simulink model "Copy_of_mcb_bldc_sixstep_f28069mLaunchPad_closeLoop"  (R2023b)
settings: Solver=FixedStepDiscrete  StartTime=0.0  StopTime=2  RelTol=1e-3  EnableMultiTasking=on
InitFcn:
  | mcb_bldc_sixstep_f28069mLaunchPad_data;
values from neighbouring files (symbols this model uses):
  bldc = mcb_SetPMSMMotorParameters('D60MR6430')    [mcb_bldc_sixstep_f28069mLaunchPad_data.m]
  inverter = mcb_SetInverterParameters('SBLMB500')    [mcb_bldc_sixstep_f28069mLaunchPad_data.m]
  PI_params = mcb_SetControllerParameters(bldc,inverter,PU_System,T_pwm,2*Ts,Ts_speed)    [mcb_bldc_sixstep_f28069mLaunchPad_data.m]
  speedRefADCOffset = 44    [mcb_bldc_sixstep_f28069mLaunchPad_data.m]
  target = mcb_SetProcessorDetails('F28069M',PWM_frequency)    [mcb_bldc_sixstep_f28069mLaunchPad_data.m]
  Ts = 0.03    [dataMonitoringArr.m]    (also in mcb_bldc_sixstep_f28069mLaunchPad_data.m = 5e-05)
  Ts_speed = 10*Ts    (= 0.0005)    [mcb_bldc_sixstep_f28069mLaunchPad_data.m]
undefined symbols (not defined in the file or in its folder): Down, GPTRIP1SEL, GPTRIP2SEL, TZ1, TZ2, Up
libraries: c2802xlib x8, c2806xlib x6, c280xlib x5, mcbcontrolslib x3, mcbpositiondecoderlib x3, slpidlib x2, simulink x2, svdschedulerlib x1
(part 2 of 2)

== system Copy_of_mcb_bldc_sixstep_f28069mLaunchPad_closeLoop/Current Control/Data_Logging/Data_Conditioning ==
  In1 : Inport
  Data Type Conversion : DataTypeConversion  OutDataTypeStr=fixdt(1,16,12)  RndMeth=Simplest  SaturateOnIntegerOverflow=off
  Data Type Conversion3 : DataTypeConversion  OutDataTypeStr=uint16  ConvertRealWorld=Stored Integer (SI)  SaturateOnIntegerOverflow=off  RndMeth=Floor
  Out1 : Outport  VectorParamsAs1DForOutWhenUnconnected=off
  wires:
  In1/1 -> Data Type Conversion/1
  Data Type Conversion3/1 -> Out1/1
  Data Type Conversion/1 -> Data Type Conversion3/1

== system Copy_of_mcb_bldc_sixstep_f28069mLaunchPad_closeLoop/Current Control/Data_Logging/End ==
  Data : Inport
  Data_width : Inport  Port=2
  Action Port : ActionPort  ActionPortLabel=elseif(u1 == 599)
  Bias : Bias  Bias=1  SaturateOnIntegerOverflow=off
  Mux : Mux  Inputs=2
  Start : Constant  Value=hex2dec('4545')  OutDataTypeStr=uint16
  Data_out : Outport  VectorParamsAs1DForOutWhenUnconnected=off
  Iteration : Outport  Port=2  VectorParamsAs1DForOutWhenUnconnected=off
  wires:
  Mux/1 -> Data_out/1
  Data_width/1 -> Bias/1
  Start/1 -> Mux/2
  Bias/1 -> Iteration/1
  Data/1 -> Mux/1

== system Copy_of_mcb_bldc_sixstep_f28069mLaunchPad_closeLoop/Current Control/Data_Logging/Start ==
  Data : Inport
  Data_width : Inport  Port=2
  Action Port : ActionPort  ActionPortLabel=if(u1 == 0)
  Bias : Bias  Bias=1  SaturateOnIntegerOverflow=off
  End : Constant  Value=hex2dec('5353')  OutDataTypeStr=uint16
  Mux : Mux  Inputs=2
  Data_out : Outport  VectorParamsAs1DForOutWhenUnconnected=off
  Iteration : Outport  Port=2  VectorParamsAs1DForOutWhenUnconnected=off
  wires:
  End/1 -> Mux/1
  Mux/1 -> Data_out/1
  Data_width/1 -> Bias/1
  Bias/1 -> Iteration/1
  Data/1 -> Mux/2

== system Copy_of_mcb_bldc_sixstep_f28069mLaunchPad_closeLoop/Current Control/Data_Transmit/CodeGeneration ==
  Input : Inport
  Add : Sum  Inputs=+-  OutDataTypeStr=Inherit: Same as first input
  Demux2 : Demux  Outputs=2
  Index Vector : MultiPortSwitch  Inputs=1  SaturateOnIntegerOverflow=off  InputSameDT=off
  SCI Transmit : c280xlib/SCI Transmit  sciModule=A  dataHead=''  dataTail=''  frameSize=1  blockingMode=on  outputStatus=off
  While Iterator : WhileIterator  MaxIters=-1  WhileBlockType=do-while  ShowIterationPort=on  OutputDataType=int16
  wires:
  While Iterator/1 -> Add/2, Index Vector/1
  Demux2/1 -> Index Vector/2
  Index Vector/1 -> SCI Transmit/1
  Add/1 -> While Iterator/1
  Demux2/2 -> Add/1
  Input/1 -> Demux2/1

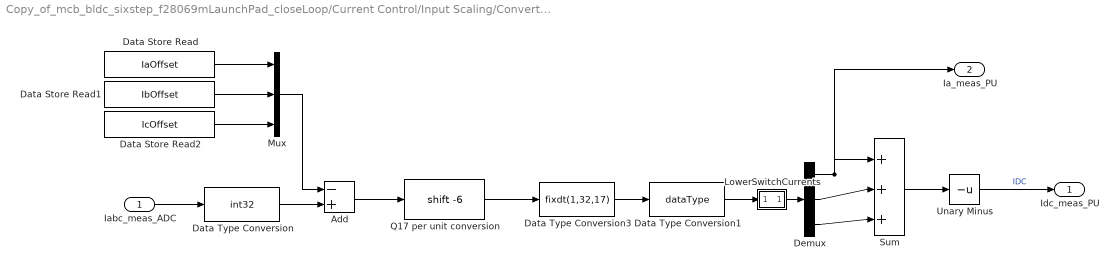
== system Copy_of_mcb_bldc_sixstep_f28069mLaunchPad_closeLoop/Current Control/Input Scaling/Convert ADC value to PU ==
  Iabc_meas_ADC : Inport
  Add : Sum  Inputs=-+
  Data Store Read : DataStoreRead  DataStoreName=IaOffset  IndexOptions=Index vector (dialog)  Indices=1  OutputSizes=1
  Data Store Read1 : DataStoreRead  DataStoreName=IbOffset  IndexOptions=Index vector (dialog)  Indices=1  OutputSizes=1
  Data Store Read2 : DataStoreRead  DataStoreName=IcOffset  IndexOptions=Index vector (dialog)  Indices=1  OutputSizes=1
  Data Type Conversion : DataTypeConversion  OutDataTypeStr=int32  ConvertRealWorld=Stored Integer (SI)  SaturateOnIntegerOverflow=off  RndMeth=Floor
  Data Type Conversion1 : DataTypeConversion  OutDataTypeStr=dataType  SaturateOnIntegerOverflow=off  RndMeth=Floor
  Data Type Conversion3 : DataTypeConversion  OutDataTypeStr=fixdt(1,32,17)  ConvertRealWorld=Stored Integer (SI)  RndMeth=Simplest  SaturateOnIntegerOverflow=off
  Demux : Demux  Outputs=3
  LowerSwitchCurrents : Subsystem
  Mux : Mux  Inputs=3
  Q17 per unit conversion : ArithShift  BitShiftNumber=-6
  Sum : Sum  Inputs=|+++
  Unary Minus : UnaryMinus
  Idc_meas_PU : Outport
  Ia_meas_PU : Outport  Port=2
  wires:
  Data Type Conversion3/1 -> Data Type Conversion1/1
  Q17 per unit conversion/1 -> Data Type Conversion3/1
  Demux/2 -> Sum/2
  Demux/1 -> Ia_meas_PU/1, Sum/1
  Sum/1 -> Unary Minus/1
  Demux/3 -> Sum/3
  Data Type Conversion1/1 -> LowerSwitchCurrents/1(in)
  Data Store Read2/1 -> Mux/3
  Data Store Read1/1 -> Mux/2
  Data Store Read/1 -> Mux/1
  Iabc_meas_ADC/1 -> Data Type Conversion/1
  Data Type Conversion/1 -> Add/2
  Mux/1 -> Add/1
  Add/1 -> Q17 per unit conversion/1
  Unary Minus/1 -> Idc_meas_PU/1  "IDC"
  LowerSwitchCurrents/1(cu) -> Demux/1

== system Copy_of_mcb_bldc_sixstep_f28069mLaunchPad_closeLoop/Current Control/Input Scaling/QEP Feedback ==
  Qep_Meas : Inport
  " Calculate Position and Speed" : Subsystem
  Demux : Demux  Outputs=2
  IndexOffset : Constant  Value=bldc.PositionOffset  OutDataTypeStr=dataType  SampleTime=-1
  speed : Outport
  Theta_e : Outport  Port=2
  wires:
  Demux/1 -> " Calculate Position and Speed"/1(QEP_Position_Count)
  IndexOffset/1 -> " Calculate Position and Speed"/3(Offset)
  Demux/2 -> " Calculate Position and Speed"/2(QEP_Index_Latch)
  " Calculate Position and Speed"/1(Theta_e) -> Theta_e/1
  Qep_Meas/1 -> Demux/1
  " Calculate Position and Speed"/2(speed) -> speed/1

== system Copy_of_mcb_bldc_sixstep_f28069mLaunchPad_closeLoop/Current Control/Sensor Driver Blocks/Convert ADC to PU ==
  ADCin : Inport
  ADCThreshold : Switch  Criteria=u2 > Threshold  Threshold=speedRefADCOffset  SaturateOnIntegerOverflow=off  InputSameDT=off
  Constant : Constant  Value=speedRefADCOffset
  LowerThreshold : Constant  Value=0
  Sum : Sum  Inputs=-|+
  Torque sign : Subsystem
  conductSpeed : Product  OutDataTypeStr=single
  toPU : Gain  Gain=1/4096  OutDataTypeStr=single
  speedPUout : Outport
  wires:
  Torque sign/1(TorqueSign) -> conductSpeed/1
  LowerThreshold/1 -> ADCThreshold/3
  toPU/1 -> conductSpeed/2
  conductSpeed/1 -> speedPUout/1
  ADCin/1 -> Sum/2, ADCThreshold/2
  ADCThreshold/1 -> toPU/1
  Constant/1 -> Sum/1
  Sum/1 -> ADCThreshold/1

== system Copy_of_mcb_bldc_sixstep_f28069mLaunchPad_closeLoop/Hardware Init/Variant Subsystem/Code Generation ==
  note: for BoostXL-DRV8305 connected to LaunchXL-28069M
  note: System Outputs
  In1 : Inport
  ADC Calib Enable : Constant  Value=inverter.ADCOffsetCalibEnable
  "Calculate ADC Offset " : Subsystem  Priority=1001  TreatAsAtomicUnit=on
  DRV Enable : Subsystem  Priority=1
  Default ADC Offset : Subsystem  Priority=1001  TreatAsAtomicUnit=on
  NOT : Logic  Operator=NOT  IconShape=distinctive  AllPortsSameDT=off  OutDataTypeStr=boolean
  wires:
  In1/1 -> DRV Enable/1(In)
  NOT/1 -> Default ADC Offset/Enable
  ADC Calib Enable/1 -> "Calculate ADC Offset "/Enable, NOT/1

== system Copy_of_mcb_bldc_sixstep_f28069mLaunchPad_closeLoop/Hardware Init/Variant Subsystem/Simulation ==
  In1 : Inport
  Terminator : Terminator
  wires:
  In1/1 -> Terminator/1

== system Copy_of_mcb_bldc_sixstep_f28069mLaunchPad_closeLoop/To_LCD/Data_Logging/Data ==
  Data : Inport
  Data_width : Inport  Port=2
  Action Port : ActionPort  ActionPortLabel=else
  Mux : Mux  Inputs=2
  Start : Constant  Value=hex2dec('0000')  OutDataTypeStr=uint16
  Data_out : Outport  VectorParamsAs1DForOutWhenUnconnected=off
  Iteration : Outport  Port=2  VectorParamsAs1DForOutWhenUnconnected=off
  wires:
  Start/1 -> Mux/2
  Mux/1 -> Data_out/1
  Data/1 -> Mux/1
  Data_width/1 -> Iteration/1

== system Copy_of_mcb_bldc_sixstep_f28069mLaunchPad_closeLoop/To_LCD/Data_Logging/Data_Conditioning ==
  rawDataIn : Inport
  convertTo_sfix16_En12 : DataTypeConversion  OutDataTypeStr=fixdt(1,16,12)  RndMeth=Simplest  SaturateOnIntegerOverflow=off
  convertTo_uint16 : DataTypeConversion  OutDataTypeStr=uint16  ConvertRealWorld=Stored Integer (SI)  SaturateOnIntegerOverflow=off  RndMeth=Floor
  convertedData : Outport  VectorParamsAs1DForOutWhenUnconnected=off
  wires:
  rawDataIn/1 -> convertTo_sfix16_En12/1
  convertTo_uint16/1 -> convertedData/1
  convertTo_sfix16_En12/1 -> convertTo_uint16/1

== system Copy_of_mcb_bldc_sixstep_f28069mLaunchPad_closeLoop/To_LCD/Data_Logging/End ==
  Data : Inport
  Data_width : Inport  Port=2
  Action Port : ActionPort  ActionPortLabel=elseif(u1 == 2)
  Bias : Bias  Bias=1  SaturateOnIntegerOverflow=off
  Mux : Mux  Inputs=2
  Start : Constant  Value=hex2dec('4545')  OutDataTypeStr=uint16
  Data_out : Outport  VectorParamsAs1DForOutWhenUnconnected=off
  Iteration : Outport  Port=2  VectorParamsAs1DForOutWhenUnconnected=off
  wires:
  Mux/1 -> Data_out/1
  Data_width/1 -> Bias/1
  Start/1 -> Mux/2
  Bias/1 -> Iteration/1
  Data/1 -> Mux/1

== system Copy_of_mcb_bldc_sixstep_f28069mLaunchPad_closeLoop/To_LCD/Data_Logging/Start ==
  Data : Inport
  Data_width : Inport  Port=2
  Action Port : ActionPort  ActionPortLabel=if(u1 == 0)
  Bias : Bias  Bias=1  SaturateOnIntegerOverflow=off
  End : Constant  Value=hex2dec('5353')  OutDataTypeStr=uint16
  Mux : Mux  Inputs=2
  Data_out : Outport  VectorParamsAs1DForOutWhenUnconnected=off
  Iteration : Outport  Port=2  VectorParamsAs1DForOutWhenUnconnected=off
  wires:
  End/1 -> Mux/1
  Mux/1 -> Data_out/1
  Data_width/1 -> Bias/1
  Bias/1 -> Iteration/1
  Data/1 -> Mux/2

== system Copy_of_mcb_bldc_sixstep_f28069mLaunchPad_closeLoop/Current Control/Input Scaling/Convert ADC value to PU/LowerSwitchCurrents ==
  in : Inport
  Constant : Constant  Value=0
  Data Type Conversion : DataTypeConversion  SaturateOnIntegerOverflow=off  RndMeth=Floor
  Switch : Switch  Criteria=u2 > Threshold  SaturateOnIntegerOverflow=off  InputSameDT=off
  cu : Outport
  wires:
  Constant/1 -> Switch/1
  in/1 -> Switch/2, Switch/3
  Switch/1 -> Data Type Conversion/1  "cu"
  Data Type Conversion/1 -> cu/1

== system Copy_of_mcb_bldc_sixstep_f28069mLaunchPad_closeLoop/Current Control/Input Scaling/QEP Feedback/ Calculate Position and Speed ==
  QEP_Position_Count : Inport
  QEP_Index_Latch : Inport  Port=2
  Offset : Inport  Port=3
  IIR Filter : mcbcontrolslib/IIR Filter  VariantControl=Low Pass Filter  VariantSelect=Low-pass  Filter_constant=0.01  advancedSettings=off  Ts=50e-6  cutOff_freq=32.1525
  Mechanical to Electrical Position : mcbpositiondecoderlib/Mechanical to Electrical Position  PolePairsInputType=Specify via dialog  NrPP=bldc.p  selectedRange=Per unit  MechOfstInputType=Input port  mechOffsetIn=0  maxAngleIn=1  InputDataType=dataType  VariantSelect=floating-point
  Quadrature Decoder : mcbpositiondecoderlib/Quadrature Decoder  EncoderSlitsPerRevolution=bldc.QEPSlits  EncoderCountsPerSlit=4  CounterSize=16 bits  ExternalIndexCount=on  PositionUnit=Per unit  PositionDataType=dataType  ParameterInputType=off  CountsPerRevInverseDataType=single
  Speed Measurement : mcbpositiondecoderlib/Speed Measurement  PositionUnit=Per unit  PositionScalingDatatype=uint32  SpeedCalculationMode=Time interval for speed calculation  SampleTimeAsync=Ts  MaximumApplicationSpeed=6000  SpeedResolution=5e-6  DelayLength=20  MaximumMeasurableSpeed=29999  MeasurableSpeedResolution=1.397e-05  SpeedUnit=Per unit based on dialog  PerUnitSpeed=PU_System.N_base  SpeedDataType=dataType
  Theta_e : Outport  VectorParamsAs1DForOutWhenUnconnected=off
  speed : Outport  Port=2  VectorParamsAs1DForOutWhenUnconnected=off
  wires:
  Speed Measurement/1 -> IIR Filter/1
  Mechanical to Electrical Position/1 -> Theta_e/1
  QEP_Position_Count/1 -> Quadrature Decoder/1
  Quadrature Decoder/1 -> Speed Measurement/1, Mechanical to Electrical Position/1
  Offset/1 -> Mechanical to Electrical Position/2
  IIR Filter/1 -> speed/1
  QEP_Index_Latch/1 -> Quadrature Decoder/2

== system Copy_of_mcb_bldc_sixstep_f28069mLaunchPad_closeLoop/Current Control/Sensor Driver Blocks/Convert ADC to PU/Torque sign ==
  Clockwise : Subsystem  TreatAsAtomicUnit=on
  Counter_Clockwise : Subsystem  TreatAsAtomicUnit=on
  Data Store Read : DataStoreRead  DataStoreName=readTorqueSign  IndexOptions=Index vector (dialog)  Indices=1  OutputSizes=1
  If1 : If  IfExpression=u1 == 0  ElseIfExpressions=u1 == 1  ShowElse=off
  Merge1 : Merge
  Sign : Signum
  TorqueSign : Outport
  wires:
  If1/2 -> Counter_Clockwise/Action
  If1/1 -> Clockwise/Action
  Clockwise/1(CW) -> Merge1/1
  Counter_Clockwise/1(CCW) -> Merge1/2
  Data Store Read/1 -> If1/1
  Merge1/1 -> Sign/1
  Sign/1 -> TorqueSign/1

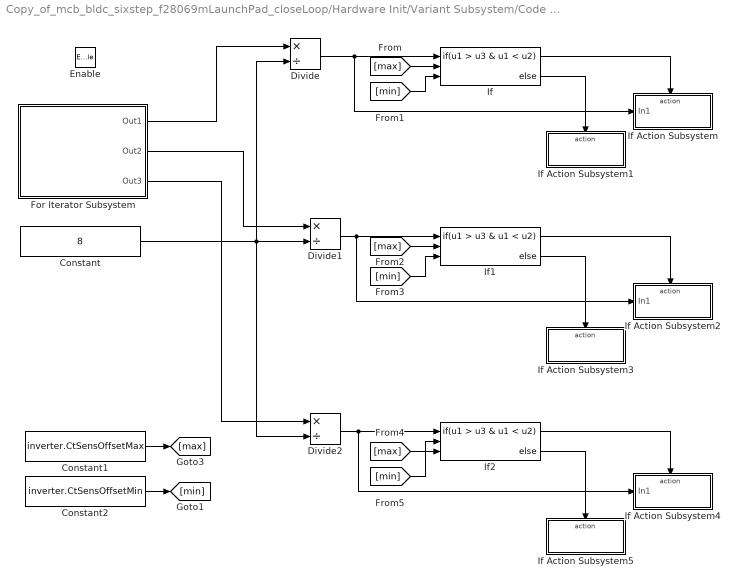
== system Copy_of_mcb_bldc_sixstep_f28069mLaunchPad_closeLoop/Hardware Init/Variant Subsystem/Code Generation/Calculate ADC Offset  ==
  Enable : EnablePort
  Constant : Constant  Value=8
  Constant1 : Constant  Value=inverter.CtSensOffsetMax  OutDataTypeStr=Inherit: Inherit via back propagation
  Constant2 : Constant  Value=inverter.CtSensOffsetMin  OutDataTypeStr=Inherit: Inherit via back propagation
  Divide : Product  Inputs=*/  OutDataTypeStr=uint16
  Divide1 : Product  Inputs=*/  OutDataTypeStr=uint16
  Divide2 : Product  Inputs=*/  OutDataTypeStr=uint16
  For Iterator Subsystem : Subsystem  TreatAsAtomicUnit=on
  If : If  NumInputs=3  IfExpression=u1 > u3 & u1 < u2
  If Action Subsystem : Subsystem  TreatAsAtomicUnit=on
  If Action Subsystem1 : Subsystem  TreatAsAtomicUnit=on
  If Action Subsystem2 : Subsystem  TreatAsAtomicUnit=on
  If Action Subsystem3 : Subsystem  TreatAsAtomicUnit=on
  If Action Subsystem4 : Subsystem  TreatAsAtomicUnit=on
  If Action Subsystem5 : Subsystem  TreatAsAtomicUnit=on
  If1 : If  NumInputs=3  IfExpression=u1 > u3 & u1 < u2
  If2 : If  NumInputs=3  IfExpression=u1 > u3 & u1 < u2
  wires:
  Divide/1 -> If Action Subsystem/1(In1), If/1
  Constant2/1 -> [min]
  [min] -> If1/3
  If2/2 -> If Action Subsystem5/Action
  [min] -> If2/3
  [max] -> If2/2
  [max] -> If1/2
  [min] -> If/3
  [max] -> If/2
  For Iterator Subsystem/1(Out1) -> Divide/1
  Constant1/1 -> [max]
  If/1 -> If Action Subsystem/Action
  If2/1 -> If Action Subsystem4/Action
  If1/1 -> If Action Subsystem2/Action
  If/2 -> If Action Subsystem1/Action
  For Iterator Subsystem/2(Out2) -> Divide1/1
  For Iterator Subsystem/3(Out3) -> Divide2/1
  If1/2 -> If Action Subsystem3/Action
  Constant/1 -> Divide2/2, Divide/2, Divide1/2
  Divide1/1 -> If1/1, If Action Subsystem2/1(In1)
  Divide2/1 -> If2/1, If Action Subsystem4/1(In1)

== system Copy_of_mcb_bldc_sixstep_f28069mLaunchPad_closeLoop/Hardware Init/Variant Subsystem/Code Generation/DRV Enable ==
  In : Inport
  DRV830x_Enable : Constant  OutDataTypeStr=Inherit: Inherit via back propagation
  Demux : Demux  Outputs=2
  Digital Output : c2806xlib/Digital Output  GPIO_Number=GPIO50~GPIO55  GPIO_Bit0=off  GPIO_BIT0_Toggle=off  GPIO_Bit1=off  GPIO_BIT1_Toggle=off  GPIO_Bit2=on  GPIO_BIT2_Toggle=off  GPIO_Bit3=off  GPIO_BIT3_Toggle=off  GPIO_Bit4=off  GPIO_BIT4_Toggle=off  GPIO_Bit5=off  GPIO_BIT5_Toggle=off  GPIO_Bit6=off  GPIO_BIT6_Toggle=off  GPIO_Bit7=off  GPIO_BIT7_Toggle=off
  Display : Display
      settings: Format=hex (Stored Integer)
  Display1 : Display
      settings: Format=hex (Stored Integer)
  SPI Master Transfer : c280xlib/SPI Controller Transfer  SPISelect=SPI_A  ClockPolarity=Rising_edge  ClockPhase=No_delay  SPIModule=uint32(0)  Mode=Master  BusSpeed=uint32(1000000)  FirstBitToTransfer=Most significant bit (MSB)  ClockMode=0  BlockFunction=Transfer  EnableRegisterAddress=off  RegisterAddress=0  OutputDataType=int8  OutputDataLength=1  DataBits=16  UseCustomSSPin=Provided by the SPI peripheral  ActiveLowSSPin=Active low  Pin=61
  SPI Master Transfer1 : c280xlib/SPI Controller Transfer  SPISelect=SPI_A  ClockPolarity=Rising_edge  ClockPhase=No_delay  SPIModule=uint32(0)  Mode=Master  BusSpeed=uint32(1000000)  FirstBitToTransfer=Most significant bit (MSB)  ClockMode=0  BlockFunction=Transfer  EnableRegisterAddress=off  RegisterAddress=0  OutputDataType=int8  OutputDataLength=1  DataBits=16  UseCustomSSPin=Provided by the SPI peripheral  ActiveLowSSPin=Active low  Pin=61
  wires:
  Demux/2 -> SPI Master Transfer1/1
  SPI Master Transfer1/1 -> Display1/1
  SPI Master Transfer/1 -> Display/1
  Demux/1 -> SPI Master Transfer/1
  In/1 -> Demux/1
  DRV830x_Enable/1 -> Digital Output/1

== system Copy_of_mcb_bldc_sixstep_f28069mLaunchPad_closeLoop/Hardware Init/Variant Subsystem/Code Generation/Default ADC Offset ==
  Enable : EnablePort
  Constant : Constant  Value=inverter.CtSensAOffset  OutDataTypeStr=Inherit: Inherit via back propagation
  Constant1 : Constant  Value=inverter.CtSensBOffset  OutDataTypeStr=Inherit: Inherit via back propagation
  Constant2 : Constant  Value=inverter.CtSensCOffset  OutDataTypeStr=Inherit: Inherit via back propagation
  Data Store Write1 : DataStoreWrite  DataStoreName=IaOffset  IndexOptions=Index vector (dialog)  Indices=1  OutputSizes=1
  Data Store Write2 : DataStoreWrite  DataStoreName=IbOffset  IndexOptions=Index vector (dialog)  Indices=1  OutputSizes=1
  Data Store Write3 : DataStoreWrite  DataStoreName=IcOffset  IndexOptions=Index vector (dialog)  Indices=1  OutputSizes=1
  wires:
  Constant/1 -> Data Store Write1/1
  Constant1/1 -> Data Store Write2/1
  Constant2/1 -> Data Store Write3/1

== system Copy_of_mcb_bldc_sixstep_f28069mLaunchPad_closeLoop/Current Control/Sensor Driver Blocks/Convert ADC to PU/Torque sign/Clockwise ==
  Action Port : ActionPort  ActionPortLabel=if(u1 == 0)
  Clockwise : Constant
  CW : Outport
  wires:
  Clockwise/1 -> CW/1

== system Copy_of_mcb_bldc_sixstep_f28069mLaunchPad_closeLoop/Current Control/Sensor Driver Blocks/Convert ADC to PU/Torque sign/Counter_Clockwise ==
  Action Port : ActionPort  ActionPortLabel=elseif(u1 == 1)
  Counter_Clockwise : Constant  Value=-1
  CCW : Outport
  wires:
  Counter_Clockwise/1 -> CCW/1

== system Copy_of_mcb_bldc_sixstep_f28069mLaunchPad_closeLoop/Hardware Init/Variant Subsystem/Code Generation/Calculate ADC Offset /For Iterator Subsystem ==
  Demux : Demux  Outputs=2
  For Iterator : ForIterator  IterationLimit=16  IterationVariableDataType=uint16
  IA/IB Measurement : c2802xlib/ADC  blkParamProc=C2000  ADCModule=1  samplingMode=Simultaneous sample mode  ADCResolution=12-bit (Single-ended input)  useSOC1=SOC0  useSOC2=SOC4_SOC5  SOCAcquisitionWindow=7  SOCTriggerSource=Software  SOCInterruptTrigger=No ADCINT  Ts=-1  dType=uint16  postInterrupt=off  interruptSel=ADCINT1  ADCINTContinuous=on  endma=off  chdma=1  conv1=ADCINA0  conv2=ADCINA0 and ADCINB0  conv1_Type4=ADCIN0  conv2_Type4=ADCIN0 and ADCIN1
  IC Measurement : c2802xlib/ADC  blkParamProc=C2000  ADCModule=1  samplingMode=Single sample mode  ADCResolution=12-bit (Single-ended input)  useSOC1=SOC3  useSOC2=SOC2_SOC3  SOCAcquisitionWindow=7  SOCTriggerSource=Software  SOCInterruptTrigger=No ADCINT  Ts=-1  dType=uint16  postInterrupt=off  interruptSel=ADCINT1  ADCINTContinuous=on  endma=off  chdma=1  conv1=ADCINA1  conv2=ADCINA1 and ADCINB1  conv1_Type4=ADCIN0  conv2_Type4=ADCIN0 and ADCIN1
  If : If  IfExpression=u1 > 8  ShowElse=off
  If Action Subsystem : Subsystem  TreatAsAtomicUnit=on
  Out1 : Outport
  Out2 : Outport  Port=2
  Out3 : Outport  Port=3
  wires:
  For Iterator/1 -> If/1
  If Action Subsystem/1(Out1) -> Out1/1
  If Action Subsystem/2(Out2) -> Out2/1
  If/1 -> If Action Subsystem/Action
  Demux/1 -> If Action Subsystem/1(In1)
  Demux/2 -> If Action Subsystem/2(In2)
  IA/IB Measurement/1 -> Demux/1
  If Action Subsystem/3(Out3) -> Out3/1
  IC Measurement/1 -> If Action Subsystem/3(In3)

== system Copy_of_mcb_bldc_sixstep_f28069mLaunchPad_closeLoop/Hardware Init/Variant Subsystem/Code Generation/Calculate ADC Offset /If Action Subsystem ==
  In1 : Inport
  Action Port : ActionPort  ActionPortLabel=if(u1 > u3 & u1 < u2)
  Data Store Write1 : DataStoreWrite  DataStoreName=IaOffset  IndexOptions=Index vector (dialog)  Indices=1  OutputSizes=1
  wires:
  In1/1 -> Data Store Write1/1

== system Copy_of_mcb_bldc_sixstep_f28069mLaunchPad_closeLoop/Hardware Init/Variant Subsystem/Code Generation/Calculate ADC Offset /If Action Subsystem1 ==
  Action Port : ActionPort  ActionPortLabel=else
  Constant : Constant  Value=inverter.CtSensAOffset  OutDataTypeStr=Inherit: Inherit via back propagation
  Data Store Write1 : DataStoreWrite  DataStoreName=IaOffset  IndexOptions=Index vector (dialog)  Indices=1  OutputSizes=1
  wires:
  Constant/1 -> Data Store Write1/1

== system Copy_of_mcb_bldc_sixstep_f28069mLaunchPad_closeLoop/Hardware Init/Variant Subsystem/Code Generation/Calculate ADC Offset /If Action Subsystem2 ==
  In1 : Inport
  Action Port : ActionPort  ActionPortLabel=if(u1 > u3 & u1 < u2)
  Data Store Write2 : DataStoreWrite  DataStoreName=IbOffset  IndexOptions=Index vector (dialog)  Indices=1  OutputSizes=1
  wires:
  In1/1 -> Data Store Write2/1

== system Copy_of_mcb_bldc_sixstep_f28069mLaunchPad_closeLoop/Hardware Init/Variant Subsystem/Code Generation/Calculate ADC Offset /If Action Subsystem3 ==
  Action Port : ActionPort  ActionPortLabel=else
  Constant1 : Constant  Value=inverter.CtSensBOffset  OutDataTypeStr=Inherit: Inherit via back propagation
  Data Store Write2 : DataStoreWrite  DataStoreName=IbOffset  IndexOptions=Index vector (dialog)  Indices=1  OutputSizes=1
  wires:
  Constant1/1 -> Data Store Write2/1

== system Copy_of_mcb_bldc_sixstep_f28069mLaunchPad_closeLoop/Hardware Init/Variant Subsystem/Code Generation/Calculate ADC Offset /If Action Subsystem4 ==
  In1 : Inport
  Action Port : ActionPort  ActionPortLabel=if(u1 > u3 & u1 < u2)
  Data Store Write2 : DataStoreWrite  DataStoreName=IcOffset  IndexOptions=Index vector (dialog)  Indices=1  OutputSizes=1
  wires:
  In1/1 -> Data Store Write2/1

== system Copy_of_mcb_bldc_sixstep_f28069mLaunchPad_closeLoop/Hardware Init/Variant Subsystem/Code Generation/Calculate ADC Offset /If Action Subsystem5 ==
  Action Port : ActionPort  ActionPortLabel=else
  Constant1 : Constant  Value=inverter.CtSensCOffset  OutDataTypeStr=Inherit: Inherit via back propagation
  Data Store Write2 : DataStoreWrite  DataStoreName=IcOffset  IndexOptions=Index vector (dialog)  Indices=1  OutputSizes=1
  wires:
  Constant1/1 -> Data Store Write2/1

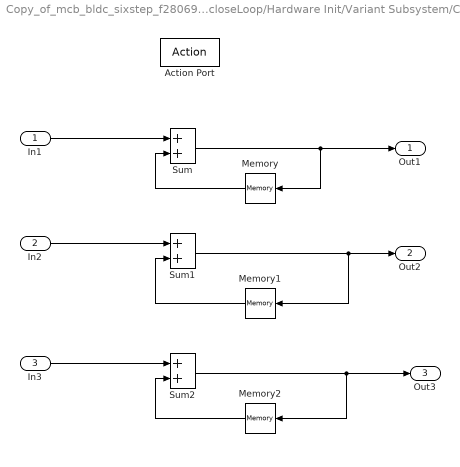
== system Copy_of_mcb_bldc_sixstep_f28069mLaunchPad_closeLoop/Hardware Init/Variant Subsystem/Code Generation/Calculate ADC Offset /For Iterator Subsystem/If Action Subsystem ==
  In1 : Inport
  In2 : Inport  Port=2
  In3 : Inport  Port=3
  Action Port : ActionPort  ActionPortLabel=if(u1 > 8)
  Memory : Memory  InheritSampleTime=on
  Memory1 : Memory  InheritSampleTime=on
  Memory2 : Memory  InheritSampleTime=on
  Sum : Sum
  Sum1 : Sum
  Sum2 : Sum
  Out1 : Outport
  Out2 : Outport  Port=2
  Out3 : Outport  Port=3
  wires:
  In1/1 -> Sum/1
  Sum/1 -> Out1/1, Memory/1
  In2/1 -> Sum1/1
  Memory/1 -> Sum/2
  Sum1/1 -> Out2/1, Memory1/1
  Memory1/1 -> Sum1/2
  In3/1 -> Sum2/1
  Sum2/1 -> Memory2/1, Out3/1
  Memory2/1 -> Sum2/2
